simulink model "pr634_phased_detector_loop_filter_vco"  (R2018b)
settings: Solver=VariableStepAuto  StartTime=0.0  StopTime=2*sim_time  RelTol=1e-3  EnableMultiTasking=on
PreLoadFcn:
  | fs=100e6;
  | sim_time=32e-5;
libraries: commsynccomp2 x2
CloseFcn:
  | clear all;
settings Model: Creator=GRIHA  LastModifiedBy=Григорий Фокин
settings DataIOCC: LimitDataPoints=on
settings OptimizationCC: LifeSpan=inf
settings DebuggingCC: AllowSymbolicDim=off  SFUnexpectedBacktrackingDiag=warning  SFNoUnconditionalDefaultTransitionDiag=warning  SFExecutionAtInitializationDiag=none
settings ModelReferenceCC: PropagateSignalLabelsOutOfModel=off
settings SFSimCC: SimUseLocalCustomCode=off
settings RTWCC: RTWUseLocalCustomCode=off
settings CodeAppCC: StateflowObjectComments=on
settings GRTTargetCC: TargetLangStandard=C89/C90 (ANSI)
settings ConfigComp: CovMetricSettings=dw  CovHtmlReporting=on  CovSaveCumulativeToWorkspaceVar=on  CovSaveSingleToWorkspaceVar=on  CovExternalEMLEnable=off

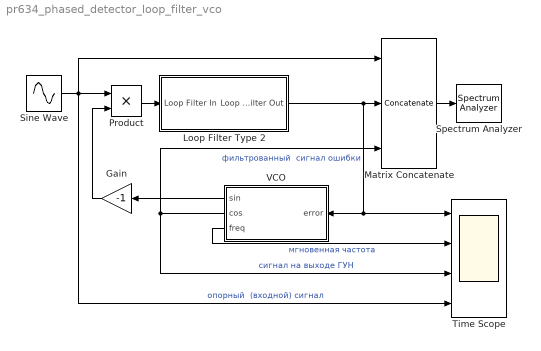
== system pr634_phased_detector_loop_filter_vco ==
  Gain : Gain  Gain=-1
  Loop Filter Type 2 : Subsystem  mask{K1=0.03125, K2=1.25e-4}
      mask prompts: K1 "K1 (proportional path)"; K2 "K2 (integral path)"
  Matrix Concatenate : Concatenate  NumInputs=3  Mode=Multidimensional array  ConcatenateDimension=2
  Product : Product
  Sine Wave : Sin  Frequency=2*pi*3.6e6  SampleTime=1/fs
  Spectrum Analyzer : SpectrumAnalyzer
  Time Scope : Scope  NumInputPorts=4
  VCO : Subsystem  mask{fr=3.5e6, sensitivity=1e6}
      mask prompts: fr "Quiescent Frequency (Hz)"; sensitivity "Sensitivity (Hz/V)"
  wires:
  Product/1 -> Loop Filter Type 2/1(Loop Filter In)
  VCO/1(sin) -> Gain/1
  Gain/1 -> Product/2
  Loop Filter Type 2/1(Loop Filter Out) -> VCO/1(error), Time Scope/1, Matrix Concatenate/2  "фильтрованный  сигнал ошибки"
  VCO/2(cos) -> Time Scope/3, Matrix Concatenate/3  "сигнал на выходе ГУН"
  Matrix Concatenate/1 -> Spectrum Analyzer/1
  VCO/3(freq) -> Time Scope/2  "мгновенная частота"
  Sine Wave/1 -> Product/1, Time Scope/4, Matrix Concatenate/1  "опорный  (входной) сигнал"

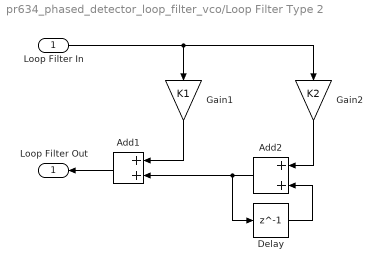
== system pr634_phased_detector_loop_filter_vco/Loop Filter Type 2 ==
  Loop Filter In : Inport
  Add1 : Sum
  Add2 : Sum
  Delay : Delay  DelayLength=1  InitialCondition=0
  Gain1 : Gain  Gain=K1
  Gain2 : Gain  Gain=K2
  Loop Filter Out : Outport
  wires:
  Loop Filter In/1 -> Gain2/1, Gain1/1
  Add1/1 -> Loop Filter Out/1
  Gain1/1 -> Add1/1
  Add2/1 -> Delay/1, Add1/2
  Gain2/1 -> Add2/1
  Delay/1 -> Add2/2

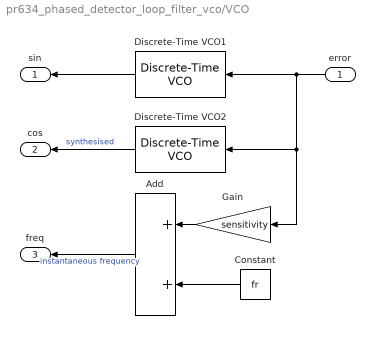
== system pr634_phased_detector_loop_filter_vco/VCO ==
  error : Inport
  Add : Sum
  Constant : Constant  Value=fr
  Discrete-Time VCO1 : commsynccomp2/Discrete-Time VCO  Ac=1  Fc=fr  Kc=sensitivity  Ph=0  ts=1/fs
      settings: SourceProductName=Communications System Toolbox  SourceProductBaseCode=CM
  Discrete-Time VCO2 : commsynccomp2/Discrete-Time VCO  Ac=1  Fc=fr  Kc=sensitivity  Ph=pi/2  ts=1/fs
      settings: SourceProductName=Communications System Toolbox  SourceProductBaseCode=CM
  Gain : Gain  Gain=sensitivity
  sin : Outport
  cos : Outport  Port=2
  freq : Outport  Port=3
  wires:
  Add/1 -> freq/1  "instantaneous frequency"
  error/1 -> Discrete-Time VCO1/1, Discrete-Time VCO2/1, Gain/1
  Discrete-Time VCO1/1 -> sin/1
  Constant/1 -> Add/2
  Discrete-Time VCO2/1 -> cos/1  "synthesised"
  Gain/1 -> Add/1
